simulink model "AKF_CT"  (Simulink 6.6)
settings: Solver=ode45  StartTime=0.0  StopTime=1.6  RelTol=1e-3
undefined symbols (not defined in the file): DiscIntNeverNeededParam
libraries: dspbuff3 x1, dspstat3 x1, commseqgen2 x1, commutil2 x1
settings Model: Creator=Home  LastModifiedBy=Мама Люда  SimulationMode=accelerator
settings OptimizationCC: InlineInvariantSignals=on
settings DebuggingCC: SignalResolutionControl=TryResolveAllWithWarning  MultiTaskDSMMsg=warning  MultiTaskCondExecSysMsg=none  StrictBusMsg=None
settings RTWCC: IncludeERTFirstTime=on

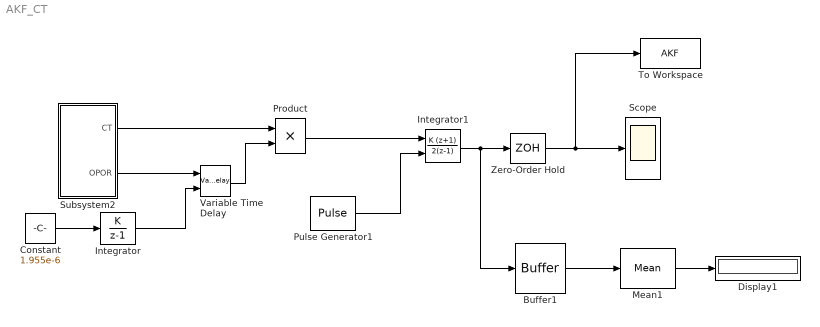
== system AKF_CT ==
  Buffer1 : dspbuff3/Buffer  N=1022  V=0  ic=0
  Constant : Constant  Value=1.955e-6  SampleTime=1e-3
  Display1 : Display
  Integrator : DiscreteIntegrator  IntegratorMethod=Accumulation: Forward Euler  gainval=1  SampleTime=1e-3  ICPrevOutput=DiscIntNeverNeededParam  ICPrevScaledInput=DiscIntNeverNeededParam
  Integrator1 : DiscreteIntegrator  IntegratorMethod=Accumulation: Trapezoidal  gainval=1/511  ExternalReset=falling  SampleTime=1.955e-6  ICPrevOutput=DiscIntNeverNeededParam  ICPrevScaledInput=DiscIntNeverNeededParam
  Mean1 : dspstat3/Mean  DialogController=dspDDGCreate  DialogControllerArgs=DataTag0  run=off  reset_popup=None  roundingMode=Floor  overflowMode=off
  Product : Product  RndMeth=Zero
  Pulse Generator1 : DiscretePulseGenerator  PulseType=Time based  Period=1e-3  PulseWidth=50  PhaseDelay=0.5e-3
  Scope : Scope
      settings: TickLabels=on  TimeRange=1  YMin=-0.05  YMax=1  SampleInput=on  SampleTime=1e-3
  Subsystem2 : Subsystem
  To Workspace : ToWorkspace  VariableName=AKF  SampleTime=1e-3  SaveFormat=Array
  Variable Time Delay : VariableTransportDelay  MaximumDelay=1024
  Zero-Order Hold : ZeroOrderHold  SampleTime=1e-3
  wires:
  Subsystem2/1(CT) -> Product/1
  Product/1 -> Integrator1/1
  Pulse Generator1/1 -> Integrator1/2
  Subsystem2/2(OPOR) -> Variable Time Delay/1
  Variable Time Delay/1 -> Product/2
  Integrator/1 -> Variable Time Delay/2
  Constant/1 -> Integrator/1
  Integrator1/1 -> Zero-Order Hold/1, Buffer1/1
  Zero-Order Hold/1 -> Scope/1, To Workspace/1
  Mean1/1 -> Display1/1
  Buffer1/1 -> Mean1/1

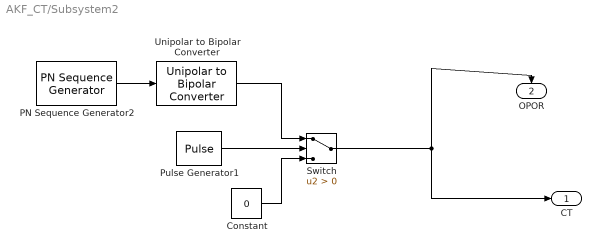
== system AKF_CT/Subsystem2 ==
  Constant : Constant  Value=0
  PN Sequence Generator2 : commseqgen2/PN Sequence Generator  poly=[9 5 0]  ini_sta=[1 1 1 1 1 1 1 1 1]  outBitMaskSource=Dialog parameter  shift=0  Ts=1.955e-6  frameBased=off  sampPerFrame=1  reset=off  bitPackedOutputs=off  outDataType=boolean  numPackedBits=8  bitPackDataSigned=off  bitPackedOutDType=double
  Pulse Generator1 : DiscretePulseGenerator  PulseType=Time based  Period=2e-3  PulseWidth=50
  Switch : Switch  Criteria=u2 > Threshold
  Unipolar to Bipolar Converter : commutil2/Unipolar to Bipolar Converter  SystemSampleTime=-1  M=2  polarity=Positive  dataType=double
  CT : Outport
  OPOR : Outport  Orientation=down  Port=2
  wires:
  PN Sequence Generator2/1 -> Unipolar to Bipolar Converter/1
  Unipolar to Bipolar Converter/1 -> Switch/1
  Pulse Generator1/1 -> Switch/2
  Switch/1 -> CT/1, OPOR/1
  Constant/1 -> Switch/3
